simulink library "RF"  (Simulink 4.00)
values from neighbouring files (symbols this model uses):
  A = rms(interp1(f,MX,fb))    [fftbandamp.m]    (also in logfft.m = fftamp(samples, fs, f, varargin{:})/vpp; plotfft.m = fftamp(samples, fs, f, varargin{:})*2/vpp)
  P = sinc((1575.42 - f)/10.23).^2./10.23    [L1PSD.m]    (also in fftphase.m = interp1(f,PX,f0))
undefined symbols (not defined in the file or in its folder): adb, B, CA_ID, fs, j, m, N, p, Phi, Range, Rice_K, Rice_Seed, Rice_Sigma, tau_delay, z
libraries: RF x133, dspcmplx x47, com_sour x8, dspelmat x8, com_chan x4, dspbdsp x3, dspswit x3, simulink_extras x2, com_filt x2
(part 3 of 5)

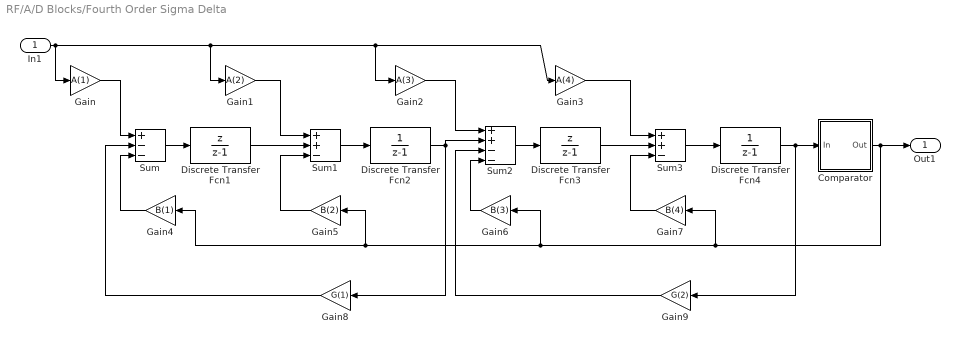
== system RF/A/D Blocks/Fourth Order Sigma Delta ==
  In1 : Inport  Port=1
  Comparator : Subsystem  mask(Comparator){L_Out=-1, H_Out=1, Bound=0}
      mask prompts: L_Out "Low Output"; H_Out "High Output"; Bound "Boundary"
      mask help: Comparator
      settings: RTWFcnNameOpts=Auto  RTWFileNameOpts=Auto
      mask Help: Outputs "low" level when the input is less than the boundary setting, and "high" when the input is above the boundary setting.
      mask Display: plot(0,0,100,100,[50,50],[0,100],[100,0],[50,50],[100,50],[70,70],[50,-0],[30,30])
  Discrete Transfer Fcn1 : DiscreteTransferFcn  Numerator=[1 0]  Denominator=[1 -1]  SampleTime=ts  Realization=auto
  Discrete Transfer Fcn2 : DiscreteTransferFcn  Numerator=[1]  Denominator=[1 -1]  SampleTime=ts  Realization=auto
  Discrete Transfer Fcn3 : DiscreteTransferFcn  Numerator=[1 0]  Denominator=[1 -1]  SampleTime=ts  Realization=auto
  Discrete Transfer Fcn4 : DiscreteTransferFcn  Numerator=[1]  Denominator=[1 -1]  SampleTime=ts  Realization=auto
  Gain : Gain  Gain=A(1)  Multiplication=Element-wise(K.*u)  SaturateOnIntegerOverflow=on
  Gain1 : Gain  Gain=A(2)  Multiplication=Element-wise(K.*u)  SaturateOnIntegerOverflow=on
  Gain2 : Gain  Gain=A(3)  Multiplication=Element-wise(K.*u)  SaturateOnIntegerOverflow=on
  Gain3 : Gain  Gain=A(4)  Multiplication=Element-wise(K.*u)  SaturateOnIntegerOverflow=on
  Gain4 : Gain  Orientation=left  Gain=B(1)  Multiplication=Element-wise(K.*u)  SaturateOnIntegerOverflow=on
  Gain5 : Gain  Orientation=left  Gain=B(2)  Multiplication=Element-wise(K.*u)  SaturateOnIntegerOverflow=on
  Gain6 : Gain  Orientation=left  Gain=B(3)  Multiplication=Element-wise(K.*u)  SaturateOnIntegerOverflow=on
  Gain7 : Gain  Orientation=left  Gain=B(4)  Multiplication=Element-wise(K.*u)  SaturateOnIntegerOverflow=on
  Gain8 : Gain  Orientation=left  Gain=G(1)  Multiplication=Element-wise(K.*u)  SaturateOnIntegerOverflow=on
  Gain9 : Gain  Orientation=left  Gain=G(2)  Multiplication=Element-wise(K.*u)  SaturateOnIntegerOverflow=on
  Sum : Sum  Inputs=+--  SaturateOnIntegerOverflow=on
  Sum1 : Sum  Inputs=++-  SaturateOnIntegerOverflow=on
  Sum2 : Sum  Inputs=++--  SaturateOnIntegerOverflow=on
  Sum3 : Sum  Inputs=++-  SaturateOnIntegerOverflow=on
  Out1 : Outport  Port=1  InitialOutput=0
  wires:
  Discrete Transfer Fcn4/1 -> Gain9/1, Comparator/1(In)
  Gain9/1 -> Sum2/3
  Gain6/1 -> Sum2/4
  Gain8/1 -> Sum/2
  Gain4/1 -> Sum/3
  Discrete Transfer Fcn2/1 -> Gain8/1, Sum2/2
  Gain2/1 -> Sum2/1
  Gain3/1 -> Sum3/1
  Gain1/1 -> Sum1/1
  Gain/1 -> Sum/1
  In1/1 -> Gain/1, Gain1/1, Gain3/1, Gain2/1
  Gain5/1 -> Sum1/3
  Gain7/1 -> Sum3/3
  Discrete Transfer Fcn3/1 -> Sum3/2
  Discrete Transfer Fcn1/1 -> Sum1/2
  Comparator/1(Out) -> Gain7/1, Gain6/1, Gain5/1, Gain4/1, Out1/1
  Sum3/1 -> Discrete Transfer Fcn4/1
  Sum/1 -> Discrete Transfer Fcn1/1
  Sum1/1 -> Discrete Transfer Fcn2/1
  Sum2/1 -> Discrete Transfer Fcn3/1

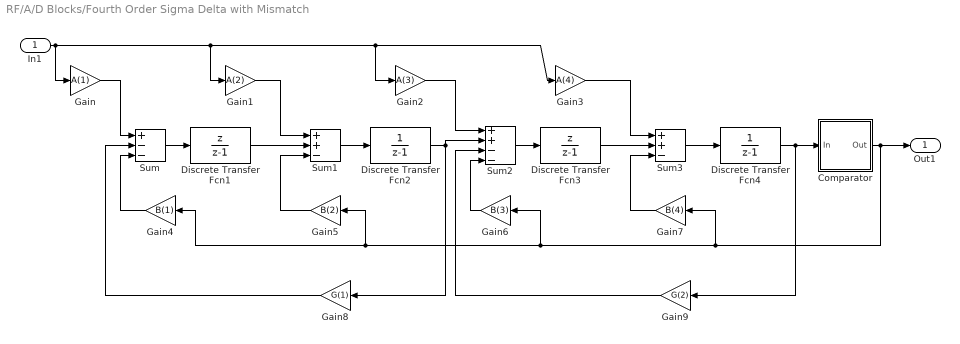
== system RF/A/D Blocks/Fourth Order Sigma Delta with Mismatch ==
  In1 : Inport  Port=1
  Comparator : Subsystem  mask(Comparator){L_Out=-1, H_Out=1, Bound=0}
      mask prompts: L_Out "Low Output"; H_Out "High Output"; Bound "Boundary"
      mask help: Comparator
      settings: RTWFcnNameOpts=Auto  RTWFileNameOpts=Auto
      mask Help: Outputs "low" level when the input is less than the boundary setting, and "high" when the input is above the boundary setting.
      mask Display: plot(0,0,100,100,[50,50],[0,100],[100,0],[50,50],[100,50],[70,70],[50,-0],[30,30])
  Discrete Transfer Fcn1 : DiscreteTransferFcn  Numerator=[1 0]  Denominator=[1 -1]  SampleTime=ts  Realization=auto
  Discrete Transfer Fcn2 : DiscreteTransferFcn  Numerator=[1]  Denominator=[1 -1]  SampleTime=ts  Realization=auto
  Discrete Transfer Fcn3 : DiscreteTransferFcn  Numerator=[1 0]  Denominator=[1 -1]  SampleTime=ts  Realization=auto
  Discrete Transfer Fcn4 : DiscreteTransferFcn  Numerator=[1]  Denominator=[1 -1]  SampleTime=ts  Realization=auto
  Gain : Gain  Gain=A(1)  Multiplication=Element-wise(K.*u)  SaturateOnIntegerOverflow=on
  Gain1 : Gain  Gain=A(2)  Multiplication=Element-wise(K.*u)  SaturateOnIntegerOverflow=on
  Gain2 : Gain  Gain=A(3)  Multiplication=Element-wise(K.*u)  SaturateOnIntegerOverflow=on
  Gain3 : Gain  Gain=A(4)  Multiplication=Element-wise(K.*u)  SaturateOnIntegerOverflow=on
  Gain4 : Gain  Orientation=left  Gain=B(1)  Multiplication=Element-wise(K.*u)  SaturateOnIntegerOverflow=on
  Gain5 : Gain  Orientation=left  Gain=B(2)  Multiplication=Element-wise(K.*u)  SaturateOnIntegerOverflow=on
  Gain6 : Gain  Orientation=left  Gain=B(3)  Multiplication=Element-wise(K.*u)  SaturateOnIntegerOverflow=on
  Gain7 : Gain  Orientation=left  Gain=B(4)  Multiplication=Element-wise(K.*u)  SaturateOnIntegerOverflow=on
  Gain8 : Gain  Orientation=left  Gain=G(1)  Multiplication=Element-wise(K.*u)  SaturateOnIntegerOverflow=on
  Gain9 : Gain  Orientation=left  Gain=G(2)  Multiplication=Element-wise(K.*u)  SaturateOnIntegerOverflow=on
  Sum : Sum  Inputs=+--  SaturateOnIntegerOverflow=on
  Sum1 : Sum  Inputs=++-  SaturateOnIntegerOverflow=on
  Sum2 : Sum  Inputs=++--  SaturateOnIntegerOverflow=on
  Sum3 : Sum  Inputs=++-  SaturateOnIntegerOverflow=on
  Out1 : Outport  Port=1  InitialOutput=0
  wires:
  Sum2/1 -> Discrete Transfer Fcn3/1
  Sum1/1 -> Discrete Transfer Fcn2/1
  Sum/1 -> Discrete Transfer Fcn1/1
  Sum3/1 -> Discrete Transfer Fcn4/1
  Comparator/1(Out) -> Out1/1, Gain4/1, Gain5/1, Gain6/1, Gain7/1
  Discrete Transfer Fcn1/1 -> Sum1/2
  Discrete Transfer Fcn3/1 -> Sum3/2
  Gain7/1 -> Sum3/3
  Gain5/1 -> Sum1/3
  In1/1 -> Gain2/1, Gain3/1, Gain1/1, Gain/1
  Gain/1 -> Sum/1
  Gain1/1 -> Sum1/1
  Gain3/1 -> Sum3/1
  Gain2/1 -> Sum2/1
  Discrete Transfer Fcn2/1 -> Sum2/2, Gain8/1
  Gain4/1 -> Sum/3
  Gain8/1 -> Sum/2
  Gain6/1 -> Sum2/4
  Gain9/1 -> Sum2/3
  Discrete Transfer Fcn4/1 -> Comparator/1(In), Gain9/1

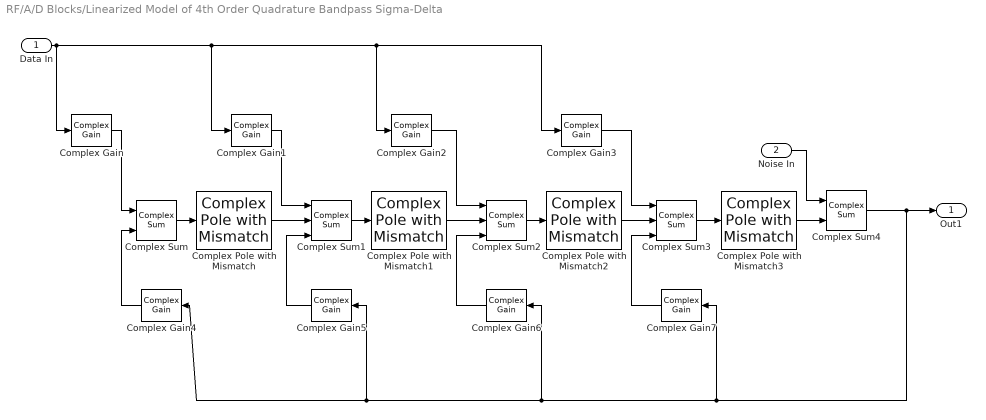
== system RF/A/D Blocks/Linearized Model of 4th Order Quadrature Bandpass Sigma-Delta ==
  Data In : Inport  Port=1
  Noise In : Inport  Port=2
  Complex Gain : RF/Complex Blocks/Complex Gain  G=a(1)+j*e(1)
  Complex Gain1 : RF/Complex Blocks/Complex Gain  G=a(2)+j*e(2)
  Complex Gain2 : RF/Complex Blocks/Complex Gain  G=a(3)+j*e(3)
  Complex Gain3 : RF/Complex Blocks/Complex Gain  G=a(4)+j*e(4)
  Complex Gain4 : RF/Complex Blocks/Complex Gain  Orientation=left  G=b(1)+j*f(1)
  Complex Gain5 : RF/Complex Blocks/Complex Gain  Orientation=left  G=b(2)+j*f(2)
  Complex Gain6 : RF/Complex Blocks/Complex Gain  Orientation=left  G=b(3)+j*f(3)
  Complex Gain7 : RF/Complex Blocks/Complex Gain  Orientation=left  G=b(4)+j*f(4)
  Complex Pole with Mismatch : RF/Complex Blocks/Complex Pole with Mismatch  c1=c1(1)  c2=c2(1)  d1=d1(1)  d2=d2(1)  ts=ts
  Complex Pole with Mismatch1 : RF/Complex Blocks/Complex Pole with Mismatch  c1=c1(2)  c2=c2(2)  d1=d1(2)  d2=d2(2)  ts=ts
  Complex Pole with Mismatch2 : RF/Complex Blocks/Complex Pole with Mismatch  c1=c1(3)  c2=c2(3)  d1=d1(3)  d2=d2(3)  ts=ts
  Complex Pole with Mismatch3 : RF/Complex Blocks/Complex Pole with Mismatch  c1=c1(4)  c2=c2(4)  d1=d1(4)  d2=d2(4)  ts=ts
  Complex Sum : dspcmplx/Complex Sum  Inputs=++
  Complex Sum1 : dspcmplx/Complex Sum  Inputs=+++
  Complex Sum2 : dspcmplx/Complex Sum  Inputs=+++
  Complex Sum3 : dspcmplx/Complex Sum  Inputs=+++
  Complex Sum4 : dspcmplx/Complex Sum  Inputs=++
  Out1 : Outport  Port=1  InitialOutput=0
  wires:
  Complex Gain4/1 -> Complex Sum/2
  Complex Pole with Mismatch/1 -> Complex Sum1/2
  Complex Sum1/1 -> Complex Pole with Mismatch1/1
  Complex Gain/1 -> Complex Sum/1
  Complex Gain1/1 -> Complex Sum1/1
  Data In/1 -> Complex Gain/1, Complex Gain1/1, Complex Gain3/1, Complex Gain2/1
  Complex Gain5/1 -> Complex Sum1/3
  Complex Sum/1 -> Complex Pole with Mismatch/1
  Complex Pole with Mismatch2/1 -> Complex Sum3/2
  Complex Pole with Mismatch1/1 -> Complex Sum2/2
  Complex Gain7/1 -> Complex Sum3/3
  Complex Gain6/1 -> Complex Sum2/3
  Complex Sum2/1 -> Complex Pole with Mismatch2/1
  Complex Gain3/1 -> Complex Sum3/1
  Complex Gain2/1 -> Complex Sum2/1
  Complex Sum3/1 -> Complex Pole with Mismatch3/1
  Complex Pole with Mismatch3/1 -> Complex Sum4/2
  Complex Sum4/1 -> Out1/1, Complex Gain7/1, Complex Gain6/1, Complex Gain5/1, Complex Gain4/1
  Noise In/1 -> Complex Sum4/1

== system RF/A/D Blocks/Second Order Simple  Lowpass  Sigma-Delta ==
  Analog_In : Inport  Port=1
  Comparator : Subsystem  mask(Comparator){L_Out=-1, H_Out=1, Bound=0}
      mask prompts: L_Out "Low Output"; H_Out "High Output"; Bound "Boundary"
      mask help: Comparator
      settings: RTWFcnNameOpts=Auto  RTWFileNameOpts=Auto
      mask Help: Outputs "low" level when the input is less than the boundary setting, and "high" when the input is above the boundary setting.
      mask Display: plot(0,0,100,100,[50,50],[0,100],[100,0],[50,50],[100,50],[70,70],[50,-0],[30,30])
  Sum : Sum  Inputs=-+  SaturateOnIntegerOverflow=on
  Sum1 : Sum  Inputs=++  SaturateOnIntegerOverflow=on
  Sum2 : Sum  Inputs=-+  SaturateOnIntegerOverflow=on
  Sum3 : Sum  Inputs=++  SaturateOnIntegerOverflow=on
  Unit Delay : UnitDelay  Orientation=left  X0=1  SampleTime=1/fs
  Unit Delay1 : UnitDelay  X0=1  SampleTime=1/fs
  Data_Out : Outport  Port=1  InitialOutput=0
  wires:
  Comparator/1(Out) -> Sum2/1, Sum/1, Data_Out/1
  Unit Delay1/1 -> Comparator/1(In), Sum3/2
  Sum2/1 -> Sum3/1
  Sum3/1 -> Unit Delay1/1
  Sum1/1 -> Sum2/2, Unit Delay/1
  Unit Delay/1 -> Sum1/2
  Analog_In/1 -> Sum/2
  Sum/1 -> Sum1/1

== system RF/A/D Blocks/Second-Order Integrator ==
  Data In : Inport  Port=1
  Discrete Filter : DiscreteFilter  Numerator=[1 zeros(1,N-1) -1]  Denominator=[1 -1]  SampleTime=1/fs  Realization=auto
  Discrete Filter1 : DiscreteFilter  Numerator=[1 zeros(1,N-1) -1]  Denominator=[1 -1]  SampleTime=1/fs  Realization=auto
  Gain : Gain  Gain=1/N  Multiplication=Element-wise(K.*u)  SaturateOnIntegerOverflow=on
  Gain1 : Gain  Gain=1/N  Multiplication=Element-wise(K.*u)  SaturateOnIntegerOverflow=on
  Data Out : Outport  Port=1  InitialOutput=0
  wires:
  Gain1/1 -> Data Out/1
  Data In/1 -> Discrete Filter/1
  Discrete Filter/1 -> Gain/1
  Discrete Filter1/1 -> Gain1/1
  Gain/1 -> Discrete Filter1/1

== system RF/A/D Blocks/Simple BandPass Sigma-Delta ==
  Analog_In : Inport  Port=1
  Comparator : RF/Circuit Models/Comparator  L_Out=-1  H_Out=1  Bound=0
  Discrete Transfer Fcn : DiscreteTransferFcn  Numerator=[-1]  Denominator="[1  0 1]"  SampleTime=1/fs  Realization=auto
  Sum : Sum  Inputs=-+  SaturateOnIntegerOverflow=on
  Data_Out : Outport  Port=1  InitialOutput=0
  wires:
  Discrete Transfer Fcn/1 -> Comparator/1
  Comparator/1 -> Sum/1, Data_Out/1
  Sum/1 -> Discrete Transfer Fcn/1
  Analog_In/1 -> Sum/2

== system RF/A/D Blocks/Simple Lowpass  Sigma-Delta ==
  Analog_In : Inport  Port=1
  Comparator : Subsystem  mask(Comparator){L_Out=-1, H_Out=1, Bound=0}
      mask prompts: L_Out "Low Output"; H_Out "High Output"; Bound "Boundary"
      mask help: Comparator
      settings: RTWFcnNameOpts=Auto  RTWFileNameOpts=Auto
      mask Help: Outputs "low" level when the input is less than the boundary setting, and "high" when the input is above the boundary setting.
      mask Display: plot(0,0,100,100,[50,50],[0,100],[100,0],[50,50],[100,50],[70,70],[50,-0],[30,30])
  Sum : Sum  Inputs=-+  SaturateOnIntegerOverflow=on
  Sum1 : Sum  Inputs=++  SaturateOnIntegerOverflow=on
  Unit Delay : UnitDelay  X0=1  SampleTime=1/fs
  Data_Out : Outport  Port=1  InitialOutput=0
  wires:
  Analog_In/1 -> Sum/2
  Comparator/1(Out) -> Data_Out/1, Sum/1
  Sum/1 -> Sum1/1
  Sum1/1 -> Unit Delay/1
  Unit Delay/1 -> Comparator/1(In), Sum1/2

== system RF/A/D Blocks/Simple Quadrature BandPass Sigma-Delta ==
  Comp_In : Inport  Port=1
  Complex Quantizer1 : RF/Complex Blocks/Complex Quantizer  L_Out_C=-1  H_Out_C=1  Bound_C=0
  Complex Resonator : Subsystem
      settings: RTWFcnNameOpts=Auto  RTWFileNameOpts=Auto
      mask Type: Complex Resonator
      mask Display: disp('Resonator')
  Complex Sum : dspcmplx/Complex Sum  Inputs=-+
  Data Out : Outport  Port=1  InitialOutput=0
  wires:
  Complex Sum/1 -> Complex Resonator/1(In1)
  Comp_In/1 -> Complex Sum/2
  Complex Quantizer1/1 -> Complex Sum/1, Data Out/1
  Complex Resonator/1(Out1) -> Complex Quantizer1/1

== system RF/A/D Blocks/Third-Order Integrator ==
  Data In : Inport  Port=1
  Discrete Filter : DiscreteFilter  Numerator=[1 zeros(1,N-1) -1]  Denominator=[1 -1]  SampleTime=1/fs  Realization=auto
  Discrete Filter1 : DiscreteFilter  Numerator=[1 zeros(1,N-1) -1]  Denominator=[1 -1]  SampleTime=1/fs  Realization=auto
  Discrete Filter2 : DiscreteFilter  Numerator=[1 zeros(1,N-1) -1]  Denominator=[1 -1]  SampleTime=1/fs  Realization=auto
  Gain : Gain  Gain=1/N  Multiplication=Element-wise(K.*u)  SaturateOnIntegerOverflow=on
  Gain1 : Gain  Gain=1/N  Multiplication=Element-wise(K.*u)  SaturateOnIntegerOverflow=on
  Gain2 : Gain  Gain=1/N  Multiplication=Element-wise(K.*u)  SaturateOnIntegerOverflow=on
  Data Out : Outport  Port=1  InitialOutput=0
  wires:
  Gain2/1 -> Data Out/1
  Gain1/1 -> Discrete Filter2/1
  Discrete Filter2/1 -> Gain2/1
  Data In/1 -> Discrete Filter/1
  Discrete Filter/1 -> Gain/1
  Discrete Filter1/1 -> Gain1/1
  Gain/1 -> Discrete Filter1/1

== system RF/Circuit Models/Clock  with Jitter ==
  Clock : Clock
      settings: DisplayTime=off  Decimation=10
  Comparator with Hysteresis : RF/Circuit Models/Comparator with Hysteresis  L_Out=VLow  H_Out=VHigh  Bound=sin(pi*(0.5-DCycle))  NPeak=PError*pi/50
  Fcn : Fcn  Expr=sin(2*pi*f0*u+Phase0)
  Gaussian noise generator : com_sour/Gaussian noise generator  m=0  d=(PError/f0/300)^2  s=Seed
  Sum : Sum  Inputs=++  SaturateOnIntegerOverflow=on
  Out1 : Outport  Port=1  InitialOutput=0
  wires:
  Fcn/1 -> Comparator with Hysteresis/1
  Comparator with Hysteresis/1 -> Out1/1
  Sum/1 -> Fcn/1
  Clock/1 -> Sum/1
  Gaussian noise generator/1 -> Sum/2

== system RF/Circuit Models/Clock  without Jitter ==
  Clock : Clock
      settings: DisplayTime=off  Decimation=10
  Comparator with Hysteresis1 : RF/Circuit Models/Comparator with Hysteresis  L_Out=VLow  H_Out=VHigh  Bound=sin(pi*(0.5-DCycle))  NPeak=PError*pi/50
  Fcn : Fcn  Expr=sin(2*pi*f0*u+Phase0)
  Out1 : Outport  Port=1  InitialOutput=0
  wires:
  Fcn/1 -> Comparator with Hysteresis1/1
  Comparator with Hysteresis1/1 -> Out1/1
  Clock/1 -> Fcn/1

== system RF/Circuit Models/Comparator ==
  In : Inport  Port=1
  Relay : Relay  OnSwitchValue=Bound  OffSwitchValue=Bound  OnOutputValue=H_Out  OffOutputValue=L_Out
  Out : Outport  Port=1  InitialOutput=0
  wires:
  Relay/1 -> Out/1
  In/1 -> Relay/1

== system RF/Circuit Models/Comparator with Hysteresis ==
  In : Inport  Port=1
  Relay : Relay  OnSwitchValue=Bound + NPeak  OffSwitchValue=Bound - NPeak  OnOutputValue=H_Out  OffOutputValue=L_Out
  Out : Outport  Port=1  InitialOutput=0
  wires:
  In/1 -> Relay/1
  Relay/1 -> Out/1

== system RF/Circuit Models/Non-Ideal Mixer ==
  RF : Inport  Port=1
  LO : Inport  Port=2
  Compression : RF/Model Nonidealities/Compression  V1dB=V1dB
  Flicker Noise : RF/Model Nonidealities/Flicker Noise  f0=f0  N0=N0  fm=fm  numtaps=numtaps  Seed=Fseed
  Nonlinear TF : RF/Model Nonidealities/Nonlinear TF  Gain1=Gain1  IIP2=IIP2  IIP3=IIP3
  Product : Product  Inputs=2  Multiplication=Element-wise(.*)  SaturateOnIntegerOverflow=on
  Saturation : Saturate  UpperLimit=1  LowerLimit=-1  LinearizeAsGain=on
  Slew Rate : RateLimiter  RisingSlewLimit=2*pi*fmax*2  FallingSlewLimit=-2*pi*fmax*2
  Sum : Sum  Inputs=++  SaturateOnIntegerOverflow=on
  White Noise : com_chan/AWGN channel  m=0  d=AWGNVRMS^2  s=SeedAWGN
  IF : Outport  Port=1  InitialOutput=0
  wires:
  RF/1 -> Product/1
  LO/1 -> Product/2
  Nonlinear TF/1 -> White Noise/1
  Product/1 -> Nonlinear TF/1
  White Noise/1 -> Sum/1
  Flicker Noise/1 -> Sum/2
  Compression/1 -> Slew Rate/1
  Slew Rate/1 -> Saturation/1
  Saturation/1 -> IF/1
  Sum/1 -> Compression/1

== system RF/Circuit Models/Non-Ideal  LNA ==
  In1 : Inport  Port=1
  Compression : RF/Model Nonidealities/Compression  V1dB=V1dB
  Flicker Noise : RF/Model Nonidealities/Flicker Noise  f0=f0  N0=N0  fm=fm  numtaps=numtaps  Seed=FSeed
  Nonlinear TF : RF/Model Nonidealities/Nonlinear TF  Gain1=Gain1  IIP2=IIP2  IIP3=IIP3
  Saturation : Saturate  UpperLimit=1  LowerLimit=-1  LinearizeAsGain=on
  Slew Rate : RateLimiter  RisingSlewLimit=2*pi*fmax*2  FallingSlewLimit=-2*pi*fmax*2
  Sum : Sum  Inputs=++  SaturateOnIntegerOverflow=on
  White Noise : com_chan/AWGN channel  m=0  d=AWGNVRMS^2  s=SeedAWGN
  Out1 : Outport  Port=1  InitialOutput=0
  wires:
  Nonlinear TF/1 -> White Noise/1
  In1/1 -> Nonlinear TF/1
  White Noise/1 -> Sum/1
  Flicker Noise/1 -> Sum/2
  Compression/1 -> Slew Rate/1
  Slew Rate/1 -> Saturation/1
  Saturation/1 -> Out1/1
  Sum/1 -> Compression/1

== system RF/Circuit Models/Quadrature Oscillator ==
  I : Sin  Amplitude=(1+AE)*A  Frequency=f0*2*pi  Phase=Phi + (pi/2 + PhiE)  SampleTime=0
  Q : Sin  Amplitude=1*A  Frequency=f0*2*pi  Phase=Phi  SampleTime=0
  Out1 : Outport  Port=1  InitialOutput=0
  Out2 : Outport  Port=2  InitialOutput=0
  wires:
  Q/1 -> Out2/1
  I/1 -> Out1/1

== system RF/Circuit Models/Simple Non-Ideal Mixer ==
  RF : Inport  Port=1
  LO : Inport  Port=2
  Nonlinear TF : RF/Model Nonidealities/Nonlinear TF  Gain1=Gain1  IIP2=IIP2  IIP3=IIP3
  Product : Product  Inputs=2  Multiplication=Element-wise(.*)  SaturateOnIntegerOverflow=on
  White Noise : com_chan/AWGN channel  m=0  d=AWGNVRMS^2  s=SeedAWGN
  IF : Outport  Port=1  InitialOutput=0
  wires:
  White Noise/1 -> IF/1
  RF/1 -> Product/1
  LO/1 -> Product/2
  Nonlinear TF/1 -> White Noise/1
  Product/1 -> Nonlinear TF/1

== system RF/Circuit Models/Simple Non-Ideal  LNA ==
  In1 : Inport  Port=1
  Nonlinear TF : RF/Model Nonidealities/Nonlinear TF  Gain1=Gain1  IIP2=IIP2  IIP3=IIP3
  White Noise : com_chan/AWGN channel  m=0  d=AWGNVRMS^2  s=SeedAWGN
  Out1 : Outport  Port=1  InitialOutput=0
  wires:
  White Noise/1 -> Out1/1
  Nonlinear TF/1 -> White Noise/1
  In1/1 -> Nonlinear TF/1

== system RF/Complex Blocks/Complex Gain ==
  In1 : Inport  Port=1
  Complex Constant : dspcmplx/Complex Constant  val=G
  Complex Multiply : dspcmplx/Complex Multiply
  Out1 : Outport  Port=1  InitialOutput=0
  wires:
  Complex Constant/1 -> Complex Multiply/2
  In1/1 -> Complex Multiply/1
  Complex Multiply/1 -> Out1/1

== system RF/Complex Blocks/Complex Quantizer ==
  In1 : Inport  Port=1
  Comparator : RF/Circuit Models/Comparator  L_Out=L_Out_C  H_Out=H_Out_C  Bound=Bound_C
  Comparator1 : RF/Circuit Models/Comparator  L_Out=L_Out_C  H_Out=H_Out_C  Bound=Bound_C
  Join : dspcmplx/Join
  Split : dspcmplx/Split
  Out1 : Outport  Port=1  InitialOutput=0
  wires:
  Split/1 -> Comparator/1
  Split/2 -> Comparator1/1
  Comparator/1 -> Join/1
  Comparator1/1 -> Join/2
  Join/1 -> Out1/1
  In1/1 -> Split/1

== system RF/Complex Blocks/Complex Unit Delay ==
  In1 : Inport  Port=1
  Join : dspcmplx/Join
  Split : dspcmplx/Split
  Unit Delay : UnitDelay  X0=icr  SampleTime=ts
  Unit Delay1 : UnitDelay  X0=ici  SampleTime=ts
  Out1 : Outport  Port=1  InitialOutput=0
  wires:
  In1/1 -> Split/1
  Join/1 -> Out1/1
  Split/2 -> Unit Delay1/1
  Split/1 -> Unit Delay/1
  Unit Delay1/1 -> Join/2
  Unit Delay/1 -> Join/1

== system RF/Complex Blocks/Complex  Continuous Pole ==
  Comp In : Inport  Port=1
  Gain1 : Gain  Orientation=left  Gain=c  Multiplication=Element-wise(K.*u)  SaturateOnIntegerOverflow=on
  Gain2 : Gain  Orientation=left  Gain=d  Multiplication=Element-wise(K.*u)  SaturateOnIntegerOverflow=on
  Gain3 : Gain  Orientation=left  Gain=c  Multiplication=Element-wise(K.*u)  SaturateOnIntegerOverflow=on
  Gain4 : Gain  Orientation=left  Gain=d  Multiplication=Element-wise(K.*u)  SaturateOnIntegerOverflow=on
  Join : dspcmplx/Join
  Split : dspcmplx/Split
  Sum : Sum  Inputs=+++  SaturateOnIntegerOverflow=on
  Sum1 : Sum  Inputs=++-  SaturateOnIntegerOverflow=on
  Transfer Fcn : TransferFcn  Numerator=[1]  Denominator=[1 0]  Realization=auto  AbsoluteTolerance=auto
  Transfer Fcn1 : TransferFcn  Numerator=[1]  Denominator=[1 0]  Realization=auto  AbsoluteTolerance=auto
  Comp Out : Outport  Port=1  InitialOutput=0
  wires:
  Comp In/1 -> Split/1
  Gain1/1 -> Sum/1
  Split/2 -> Sum/2
  Split/1 -> Sum1/2
  Gain3/1 -> Sum1/3
  Join/1 -> Comp Out/1
  Sum/1 -> Transfer Fcn/1
  Sum1/1 -> Transfer Fcn1/1
  Transfer Fcn/1 -> Gain3/1, Join/2, Gain2/1
  Transfer Fcn1/1 -> Gain1/1, Join/1, Gain4/1
  Gain2/1 -> Sum/3
  Gain4/1 -> Sum1/1

== system RF/Complex Blocks/Complex Continuous Pole with Mismatch  ==
  Comp In : Inport  Port=1
  Gain1 : Gain  Orientation=left  Gain=c2  Multiplication=Element-wise(K.*u)  SaturateOnIntegerOverflow=on
  Gain2 : Gain  Orientation=left  Gain=d2  Multiplication=Element-wise(K.*u)  SaturateOnIntegerOverflow=on
  Gain3 : Gain  Orientation=left  Gain=c1  Multiplication=Element-wise(K.*u)  SaturateOnIntegerOverflow=on
  Gain4 : Gain  Orientation=left  Gain=d1  Multiplication=Element-wise(K.*u)  SaturateOnIntegerOverflow=on
  Join : dspcmplx/Join
  Split : dspcmplx/Split
  Sum : Sum  Inputs=+++  SaturateOnIntegerOverflow=on
  Sum1 : Sum  Inputs=++-  SaturateOnIntegerOverflow=on
  Transfer Fcn : TransferFcn  Numerator=[1]  Denominator=[1 0]  Realization=auto  AbsoluteTolerance=auto
  Transfer Fcn1 : TransferFcn  Numerator=[1]  Denominator=[1 0]  Realization=auto  AbsoluteTolerance=auto
  Comp Out : Outport  Port=1  InitialOutput=0
  wires:
  Gain4/1 -> Sum1/1
  Gain2/1 -> Sum/3
  Transfer Fcn1/1 -> Gain4/1, Join/1, Gain1/1
  Transfer Fcn/1 -> Gain2/1, Join/2, Gain3/1
  Sum1/1 -> Transfer Fcn1/1
  Sum/1 -> Transfer Fcn/1
  Join/1 -> Comp Out/1
  Gain3/1 -> Sum1/3
  Split/1 -> Sum1/2
  Split/2 -> Sum/2
  Gain1/1 -> Sum/1
  Comp In/1 -> Split/1

== system RF/Complex Blocks/Complex Pole ==
  Comp In : Inport  Port=1
  Discrete Transfer Fcn : DiscreteTransferFcn  Numerator=[1]  Denominator=[1 -1]  SampleTime=ts  Realization=auto
  Discrete Transfer Fcn1 : DiscreteTransferFcn  Numerator=[1]  Denominator=[1 -1]  SampleTime=ts  Realization=auto
  Gain : Gain  Orientation=left  Gain=d  Multiplication=Element-wise(K.*u)  SaturateOnIntegerOverflow=on
  Gain1 : Gain  Orientation=left  Gain=c  Multiplication=Element-wise(K.*u)  SaturateOnIntegerOverflow=on
  Gain2 : Gain  Orientation=left  Gain=c  Multiplication=Element-wise(K.*u)  SaturateOnIntegerOverflow=on
  Gain3 : Gain  Orientation=left  Gain=d  Multiplication=Element-wise(K.*u)  SaturateOnIntegerOverflow=on
  Join : dspcmplx/Join
  Split : dspcmplx/Split
  Sum : Sum  Inputs=++-  SaturateOnIntegerOverflow=on
  Sum1 : Sum  Inputs=+++  SaturateOnIntegerOverflow=on
  Comp Out : Outport  Port=1  InitialOutput=0
  wires:
  Sum1/1 -> Discrete Transfer Fcn1/1
  Sum/1 -> Discrete Transfer Fcn/1
  Gain1/1 -> Sum/3
  Gain/1 -> Sum/1
  Gain2/1 -> Sum1/1
  Gain3/1 -> Sum1/3
  Discrete Transfer Fcn1/1 -> Gain1/1, Gain3/1, Join/2
  Discrete Transfer Fcn/1 -> Gain2/1, Gain/1, Join/1
  Comp In/1 -> Split/1
  Split/1 -> Sum/2
  Split/2 -> Sum1/2
  Join/1 -> Comp Out/1

== system RF/Complex Blocks/Complex Pole with Mismatch ==
  Comp In : Inport  Port=1
  Discrete Transfer Fcn : DiscreteTransferFcn  Numerator=[1]  Denominator=[1 -1]  SampleTime=ts  Realization=auto
  Discrete Transfer Fcn1 : DiscreteTransferFcn  Numerator=[1]  Denominator=[1 -1]  SampleTime=ts  Realization=auto
  Gain : Gain  Orientation=left  Gain=d1  Multiplication=Element-wise(K.*u)  SaturateOnIntegerOverflow=on
  Gain1 : Gain  Orientation=left  Gain=c1  Multiplication=Element-wise(K.*u)  SaturateOnIntegerOverflow=on
  Gain2 : Gain  Orientation=left  Gain=c2  Multiplication=Element-wise(K.*u)  SaturateOnIntegerOverflow=on
  Gain3 : Gain  Orientation=left  Gain=d2  Multiplication=Element-wise(K.*u)  SaturateOnIntegerOverflow=on
  Join : dspcmplx/Join
  Split : dspcmplx/Split
  Sum : Sum  Inputs=++-  SaturateOnIntegerOverflow=on
  Sum1 : Sum  Inputs=+++  SaturateOnIntegerOverflow=on
  Comp Out : Outport  Port=1  InitialOutput=0
  wires:
  Sum1/1 -> Discrete Transfer Fcn1/1
  Sum/1 -> Discrete Transfer Fcn/1
  Gain1/1 -> Sum/3
  Gain/1 -> Sum/1
  Gain2/1 -> Sum1/1
  Gain3/1 -> Sum1/3
  Discrete Transfer Fcn1/1 -> Gain1/1, Gain3/1, Join/2
  Discrete Transfer Fcn/1 -> Gain2/1, Gain/1, Join/1
  Comp In/1 -> Split/1
  Split/1 -> Sum/2
  Split/2 -> Sum1/2
  Join/1 -> Comp Out/1

== system RF/Complex Blocks/Complex Random  Number ==
  Join : dspcmplx/Join
  Random Number : RandomNumber  Mean=Mean  Variance=Sigma  Seed=Seeds(2)  SampleTime=0
  Random Number1 : RandomNumber  Mean=Mean  Variance=Sigma  Seed=Seeds(1)  SampleTime=0
  Out1 : Outport  Port=1  InitialOutput=0
  wires:
  Join/1 -> Out1/1
  Random Number1/1 -> Join/1
  Random Number/1 -> Join/2

== system RF/Filters/Butterworth BP Filter ==
  In1 : Inport  Port=1
  Butterworth BP Filter : ZeroPole  Zeros=z  Poles=p  Gain=k  AbsoluteTolerance=auto
  Out1 : Outport  Port=1  InitialOutput=0
  wires:
  In1/1 -> Butterworth BP Filter/1
  Butterworth BP Filter/1 -> Out1/1

== system RF/Filters/Butterworth BP Filter with Mismatch ==
  In1 : Inport  Port=1
  Butterworth BP Filter : ZeroPole  Zeros=z  Poles=p  Gain=k  AbsoluteTolerance=auto
  Out1 : Outport  Port=1  InitialOutput=0
  wires:
  Butterworth BP Filter/1 -> Out1/1
  In1/1 -> Butterworth BP Filter/1

== system RF/Filters/Butterworth BS Filter ==
  In1 : Inport  Port=1
  Butterworth BS Filter : ZeroPole  Zeros=z  Poles=p  Gain=k  AbsoluteTolerance=auto
  Out1 : Outport  Port=1  InitialOutput=0
  wires:
  Butterworth BS Filter/1 -> Out1/1
  In1/1 -> Butterworth BS Filter/1

== system RF/Filters/Butterworth BS Filter with Mismatch ==
  In1 : Inport  Port=1
  Butterworth BS Filter : ZeroPole  Zeros=z  Poles=p  Gain=k  AbsoluteTolerance=auto
  Out1 : Outport  Port=1  InitialOutput=0
  wires:
  In1/1 -> Butterworth BS Filter/1
  Butterworth BS Filter/1 -> Out1/1

== system RF/Filters/Butterworth HP Filter ==
  In1 : Inport  Port=1
  Butterworth HP Filter : ZeroPole  Zeros=z  Poles=p  Gain=k  AbsoluteTolerance=auto
  Out1 : Outport  Port=1  InitialOutput=0
  wires:
  Butterworth HP Filter/1 -> Out1/1
  In1/1 -> Butterworth HP Filter/1

== system RF/Filters/Butterworth HP Filter with Mismatch ==
  In1 : Inport  Port=1
  Butterworth HP Filter : ZeroPole  Zeros=z  Poles=p  Gain=k  AbsoluteTolerance=auto
  Out1 : Outport  Port=1  InitialOutput=0
  wires:
  In1/1 -> Butterworth HP Filter/1
  Butterworth HP Filter/1 -> Out1/1

== system RF/Filters/Butterworth LP Filter ==
  In1 : Inport  Port=1
  Butterworth LP Filter : ZeroPole  Zeros=z  Poles=p  Gain=k  AbsoluteTolerance=auto
  Out1 : Outport  Port=1  InitialOutput=0
  wires:
  In1/1 -> Butterworth LP Filter/1
  Butterworth LP Filter/1 -> Out1/1

== system RF/Filters/Butterworth LP Filter with Mismatch ==
  In1 : Inport  Port=1
  Butterworth LP Filter : ZeroPole  Zeros=z  Poles=p  Gain=k  AbsoluteTolerance=auto
  Out1 : Outport  Port=1  InitialOutput=0
  wires:
  Butterworth LP Filter/1 -> Out1/1
  In1/1 -> Butterworth LP Filter/1

== system RF/Filters/Chebychev Type I BP Filter ==
  In1 : Inport  Port=1
  Chebychev Type I BP Filter : ZeroPole  Zeros=z  Poles=p  Gain=k  AbsoluteTolerance=auto
  Out1 : Outport  Port=1  InitialOutput=0
  wires:
  Chebychev Type I BP Filter/1 -> Out1/1
  In1/1 -> Chebychev Type I BP Filter/1

== system RF/Filters/Chebychev Type I BP Filter with Mismatch ==
  In1 : Inport  Port=1
  Chebychev Type I BP Filter : ZeroPole  Zeros=z  Poles=p  Gain=k  AbsoluteTolerance=auto
  Out1 : Outport  Port=1  InitialOutput=0
  wires:
  In1/1 -> Chebychev Type I BP Filter/1
  Chebychev Type I BP Filter/1 -> Out1/1

== system RF/Filters/Chebychev Type I BS Filter ==
  In1 : Inport  Port=1
  Chebychev Type I BS Filter : ZeroPole  Zeros=z  Poles=p  Gain=k  AbsoluteTolerance=auto
  Out1 : Outport  Port=1  InitialOutput=0
  wires:
  Chebychev Type I BS Filter/1 -> Out1/1
  In1/1 -> Chebychev Type I BS Filter/1

== system RF/Filters/Chebychev Type I BS Filter with Mismatch ==
  In1 : Inport  Port=1
  Chebychev Type I BS Filter : ZeroPole  Zeros=z  Poles=p  Gain=k  AbsoluteTolerance=auto
  Out1 : Outport  Port=1  InitialOutput=0
  wires:
  In1/1 -> Chebychev Type I BS Filter/1
  Chebychev Type I BS Filter/1 -> Out1/1

== system RF/Filters/Chebychev Type I HP Filter ==
  In1 : Inport  Port=1
  Chebychev Type I HP Filter : ZeroPole  Zeros=z  Poles=p  Gain=k  AbsoluteTolerance=auto
  Out1 : Outport  Port=1  InitialOutput=0
  wires:
  In1/1 -> Chebychev Type I HP Filter/1
  Chebychev Type I HP Filter/1 -> Out1/1

== system RF/Filters/Chebychev Type I HP Filter with Mismatch ==
  In1 : Inport  Port=1
  Chebychev Type I HP Filter : ZeroPole  Zeros=z  Poles=p  Gain=k  AbsoluteTolerance=auto
  Out1 : Outport  Port=1  InitialOutput=0
  wires:
  Chebychev Type I HP Filter/1 -> Out1/1
  In1/1 -> Chebychev Type I HP Filter/1

== system RF/Filters/Chebychev Type I LP Filter ==
  In1 : Inport  Port=1
  Chebychev Type I LP Filter : ZeroPole  Zeros=z  Poles=p  Gain=k  AbsoluteTolerance=auto
  Out1 : Outport  Port=1  InitialOutput=0
  wires:
  Chebychev Type I LP Filter/1 -> Out1/1
  In1/1 -> Chebychev Type I LP Filter/1

== system RF/Filters/Chebychev Type I LP Filter with Mismatch ==
  In1 : Inport  Port=1
  Chebychev Type I LP Filter : ZeroPole  Zeros=z  Poles=p  Gain=k  AbsoluteTolerance=auto
  Out1 : Outport  Port=1  InitialOutput=0
  wires:
  In1/1 -> Chebychev Type I LP Filter/1
  Chebychev Type I LP Filter/1 -> Out1/1

== system RF/Filters/Complex  Image-Reject  Filter ==
  In : Inport  Port=1
  Complex Gain : RF/Complex Blocks/Complex Gain  G=A
  Complex  Continuous Pole : RF/Complex Blocks/Complex  Continuous Pole  d=d(1)  c=c(1)
  Complex  Continuous Pole1 : RF/Complex Blocks/Complex  Continuous Pole  d=d(2)  c=c(2)
  Complex  Continuous Pole2 : RF/Complex Blocks/Complex  Continuous Pole  d=d(3)  c=c(3)
  Complex  Continuous Pole3 : RF/Complex Blocks/Complex  Continuous Pole  d=d(4)  c=c(4)
  Out : Outport  Port=1  InitialOutput=0
  wires:
  Complex  Continuous Pole/1 -> Complex  Continuous Pole1/1
  Complex  Continuous Pole1/1 -> Complex  Continuous Pole2/1
  Complex  Continuous Pole2/1 -> Complex  Continuous Pole3/1
  Complex  Continuous Pole3/1 -> Out/1
  Complex Gain/1 -> Complex  Continuous Pole/1
  In/1 -> Complex Gain/1

== system RF/Filters/Complex  Image-Reject  Filter with Mismatch ==
  In : Inport  Port=1
  Complex Gain : RF/Complex Blocks/Complex Gain  G=A
  "Complex Continuous Pole with Mismatch " : RF/Complex Blocks/Complex Continuous Pole with Mismatch   c1=c1(1)  c2=c2(1)  d1=d1(1)  d2=d2(1)
  Complex Continuous Pole with Mismatch 1 : RF/Complex Blocks/Complex Continuous Pole with Mismatch   c1=c1(2)  c2=c2(2)  d1=d1(2)  d2=d2(2)
  Complex Continuous Pole with Mismatch 2 : RF/Complex Blocks/Complex Continuous Pole with Mismatch   c1=c1(3)  c2=c2(3)  d1=d1(3)  d2=d2(3)
  Complex Continuous Pole with Mismatch 3 : RF/Complex Blocks/Complex Continuous Pole with Mismatch   c1=c1(4)  c2=c2(4)  d1=d1(4)  d2=d2(4)
  Out : Outport  Port=1  InitialOutput=0
  wires:
  In/1 -> Complex Gain/1
  Complex Gain/1 -> "Complex Continuous Pole with Mismatch "/1
  "Complex Continuous Pole with Mismatch "/1 -> Complex Continuous Pole with Mismatch 1/1
  Complex Continuous Pole with Mismatch 1/1 -> Complex Continuous Pole with Mismatch 2/1
  Complex Continuous Pole with Mismatch 3/1 -> Out/1
  Complex Continuous Pole with Mismatch 2/1 -> Complex Continuous Pole with Mismatch 3/1

== system RF/Filters/RF Filter ==
  In1 : Inport  Port=1
  Transfer Fcn : TransferFcn  Numerator=num  Denominator=denom  Realization=auto  AbsoluteTolerance=auto
  Out1 : Outport  Port=1  InitialOutput=0
  wires:
  In1/1 -> Transfer Fcn/1
  Transfer Fcn/1 -> Out1/1

== system RF/GPS Blocks/C/A Code, 1.023MHz ==
  note: C/A Code Generator
  Adder : Logic  Operator=XOR  Inputs=3
  CA ID : Constant  Value=CA_PRN_ID
  Look-Up Table : Lookup  InputValues=[1:32]  OutputValues=[2;3;4;5;1;2;1;2;3;2;3;5;6;7;8;9;1;2;3;4;5;6;1;4;5;6;7;8;1;2;3;4]
  Look-Up Table1 : Lookup  InputValues=[1:32]  OutputValues=[6;7;8;9;9;10;8;9;10;3;4;6;7;8;9;10;4;5;6;7;8;9;3;6;7;8;9;10;6;7;8;9]
  PN1 : Subsystem  mask(PN(10) Sequence [3,10]){}
      mask help: Pseudo Noise Sequence (M=2^10 - 1, Feedback[3,10])
      mask init:
      | [x,y]=srcsicon(5);
      settings: RTWFcnNameOpts=Auto  RTWFileNameOpts=Auto
      mask Help: Maximal length pseudo-noise sequence with 10 memory elements.  Feedback is from taps 3 and 10.  Only the 10th tap is output.
      mask Display: plot(0,0,100,100,x,y);disp('PN Sequence ')
  PN2 : Subsystem  mask(PN(10) Sequence [2,3,6,8,9,10]){}
      mask help: Pseudo Noise Sequence (M=2^10 - 1, Feedback[2,3,6,8,9,10])
      mask init:
      | [x,y]=srcsicon(5);
      settings: RTWFcnNameOpts=Auto  RTWFileNameOpts=Auto
      mask Help: Maximal length pseudo-noise sequence with 10 memory elements.  Feedback is from taps 2, 3, 6, 8, 9,  and 10.  All phases are output.
      mask Display: plot(0,0,100,100,x,y);disp('PN Sequence\nAll Phases')
  Phase 1  Select : MultiPortSwitch  Inputs=10
  Phase 2 Select : MultiPortSwitch  Inputs=10
  Out1 : Outport  Port=1  InitialOutput=0
  wires:
  Adder/1 -> Out1/1
  Phase 2 Select/1 -> Adder/3
  PN1/1(Tap10) -> Adder/1
  Phase 1  Select/1 -> Adder/2
  PN2/10(Tap10) -> Phase 2 Select/11, Phase 1  Select/11
  PN2/9(Tap9) -> Phase 2 Select/10, Phase 1  Select/10
  PN2/8(Tap8) -> Phase 2 Select/9, Phase 1  Select/9
  PN2/7(Tap7) -> Phase 2 Select/8, Phase 1  Select/8
  PN2/6(Tap6) -> Phase 2 Select/7, Phase 1  Select/7
  PN2/5(Tap5) -> Phase 2 Select/6, Phase 1  Select/6
  PN2/4(Tap4) -> Phase 2 Select/5, Phase 1  Select/5
  PN2/3(Tap3) -> Phase 2 Select/4, Phase 1  Select/4
  PN2/2(Tap2) -> Phase 2 Select/3, Phase 1  Select/3
  PN2/1(Tap1) -> Phase 2 Select/2, Phase 1  Select/2
  Look-Up Table1/1 -> Phase 2 Select/1
  Look-Up Table/1 -> Phase 1  Select/1
  CA ID/1 -> Look-Up Table/1, Look-Up Table1/1

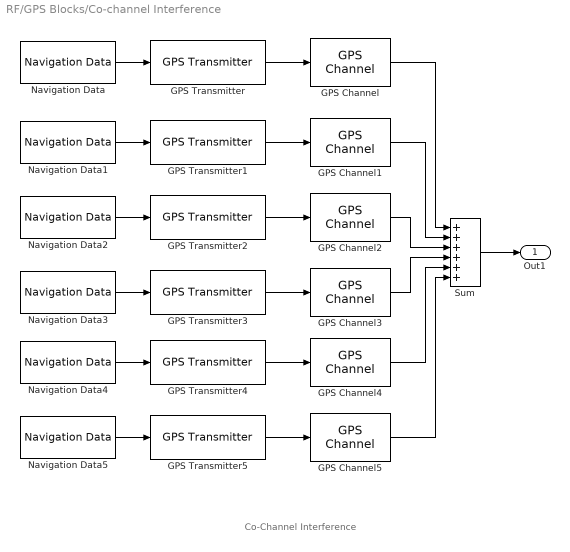
== system RF/GPS Blocks/Co-channel Interference ==
  note: Co-Channel Interference
  GPS Channel : RF/GPS Blocks/GPS Channel  Rice_Seed=Rice_Seeds(1)  tau_delay=taus_delay(1)  AWGN_Seed=AWGN_Seeds(1)  d=d(1)  tau=taus(1)
  GPS Channel1 : RF/GPS Blocks/GPS Channel  Rice_Seed=Rice_Seeds(2)  tau_delay=taus_delay(2)  AWGN_Seed=AWGN_Seeds(2)  d=d(2)  tau=taus(2)
  GPS Channel2 : RF/GPS Blocks/GPS Channel  Rice_Seed=Rice_Seeds(3)  tau_delay=taus_delay(3)  AWGN_Seed=AWGN_Seeds(3)  d=d(3)  tau=taus(3)
  GPS Channel3 : RF/GPS Blocks/GPS Channel  Rice_Seed=Rice_Seeds(4)  tau_delay=taus_delay(4)  AWGN_Seed=AWGN_Seeds(4)  d=d(4)  tau=taus(4)
  GPS Channel4 : RF/GPS Blocks/GPS Channel  Rice_Seed=Rice_Seeds(5)  tau_delay=taus_delay(5)  AWGN_Seed=AWGN_Seeds(5)  d=d(5)  tau=taus(5)
  GPS Channel5 : RF/GPS Blocks/GPS Channel  Rice_Seed=Rice_Seeds(6)  tau_delay=taus_delay(6)  AWGN_Seed=AWGN_Seeds(6)  d=d(6)  tau=taus(6)
  GPS Transmitter : RF/GPS Blocks/GPS Transmitter  tsrf=-1  CA_ID=CA(1)  P_Seed=P(1)
  GPS Transmitter1 : RF/GPS Blocks/GPS Transmitter  tsrf=-1  CA_ID=CA(2)  P_Seed=P(2)
  GPS Transmitter2 : RF/GPS Blocks/GPS Transmitter  tsrf=-1  CA_ID=CA(3)  P_Seed=P(3)
  GPS Transmitter3 : RF/GPS Blocks/GPS Transmitter  tsrf=-1  CA_ID=CA(3)  P_Seed=P(3)
  GPS Transmitter4 : RF/GPS Blocks/GPS Transmitter  tsrf=-1  CA_ID=CA(4)  P_Seed=P(4)
  GPS Transmitter5 : RF/GPS Blocks/GPS Transmitter  tsrf=-1  CA_ID=CA(5)  P_Seed=P(5)
  Navigation Data : RF/GPS Blocks/Navigation Data  Seed=Seeds(1)
  Navigation Data1 : RF/GPS Blocks/Navigation Data  Seed=Seeds(2)
  Navigation Data2 : RF/GPS Blocks/Navigation Data  Seed=Seeds(3)
  Navigation Data3 : RF/GPS Blocks/Navigation Data  Seed=Seeds(4)
  Navigation Data4 : RF/GPS Blocks/Navigation Data  Seed=Seeds(5)
  Navigation Data5 : RF/GPS Blocks/Navigation Data  Seed=Seeds(6)
  Sum : Sum  Inputs=++++++  SaturateOnIntegerOverflow=on
  Out1 : Outport  Port=1  InitialOutput=0
  wires:
  GPS Channel3/1 -> Sum/4
  GPS Channel4/1 -> Sum/5
  GPS Channel5/1 -> Sum/6
  GPS Channel2/1 -> Sum/3
  GPS Channel1/1 -> Sum/2
  GPS Channel/1 -> Sum/1
  Sum/1 -> Out1/1
  GPS Transmitter4/1 -> GPS Channel4/1
  Navigation Data4/1 -> GPS Transmitter4/1
  GPS Transmitter5/1 -> GPS Channel5/1
  Navigation Data5/1 -> GPS Transmitter5/1
  GPS Transmitter/1 -> GPS Channel/1
  Navigation Data/1 -> GPS Transmitter/1
  GPS Transmitter1/1 -> GPS Channel1/1
  Navigation Data1/1 -> GPS Transmitter1/1
  GPS Transmitter2/1 -> GPS Channel2/1
  Navigation Data2/1 -> GPS Transmitter2/1
  GPS Transmitter3/1 -> GPS Channel3/1
  Navigation Data3/1 -> GPS Transmitter3/1

== system RF/GPS Blocks/Direct Conversion Receiver ==
  note: Direct Conversion
  RF In : Inport  Port=1
  5th Order Decimation Filter : RF/A//D Blocks/5th Order Decimation Filter  N=32  fs=1E6
  5th Order Decimation Filter1 : RF/A//D Blocks/5th Order Decimation Filter  N=32  fs=1E6
  Butterworth LP Filter with Mismatch : RF/Filters/Butterworth LP Filter with Mismatch  w0=100*2*pi  order=4  ErrorStd=1
  Butterworth LP Filter with Mismatch1 : RF/Filters/Butterworth LP Filter with Mismatch  w0=100*2*pi  order=4  ErrorStd=1
  Fourth Order Sigma Delta with Mismatch : RF/A//D Blocks/Fourth Order Sigma Delta with Mismatch  NTF_Poles=p  NTF_Zeros=z  STF_Zeros=[inf inf inf]  STF_Gain=0.85  ErrorStd=1  fs=64E6
  Fourth Order Sigma Delta with Mismatch1 : RF/A//D Blocks/Fourth Order Sigma Delta with Mismatch  NTF_Poles=p  NTF_Zeros=z  STF_Zeros=[inf inf inf]  STF_Gain=0.85  ErrorStd=1  fs=64E6
  Join : dspcmplx/Join
  Non-Ideal Mixer : RF/Circuit Models/Non-Ideal Mixer  Gain1=0  IIP2=40  IIP3=40  fmax=1200  V1dB=-4  AWGNVRMS=1E-12  SeedAWGN=1  Fseed=2  f0=1000  N0=1.147E-7  fm=10E3  numtaps=100
  Non-Ideal Mixer1 : RF/Circuit Models/Non-Ideal Mixer  Gain1=0  IIP2=40  IIP3=40  fmax=1200  V1dB=-4  AWGNVRMS=1E-12  SeedAWGN=1  Fseed=2  f0=1000  N0=1.147E-7  fm=10E3  numtaps=100
  Non-Ideal  LNA : RF/Circuit Models/Non-Ideal  LNA  Gain1=0  IIP2=30  IIP3=20  AWGNVRMS=1E-3  fmax=3E9  V1dB=-4  SeedAWGN=123  FSeed=2  f0=1000  N0=1.147E-7  fm=10E3  numtaps=100
  Quadrature Oscillator : RF/Circuit Models/Quadrature Oscillator  PhiE=deg2rad(2)  AE=adb(0.1)  Phi=0  A=1  f0=1575.42E6
  RF Filter : RF/Filters/RF Filter  Q=5  f0=1575.42E6  n=1  Gi=1
  Data Out : Outport  Port=1  InitialOutput=0
  wires:
  Non-Ideal  LNA/1 -> Non-Ideal Mixer/2, Non-Ideal Mixer1/1
  RF Filter/1 -> Non-Ideal  LNA/1
  RF In/1 -> RF Filter/1
  Non-Ideal Mixer/1 -> Butterworth LP Filter with Mismatch/1
  Butterworth LP Filter with Mismatch/1 -> Fourth Order Sigma Delta with Mismatch/1
  Fourth Order Sigma Delta with Mismatch/1 -> 5th Order Decimation Filter/1
  Non-Ideal Mixer1/1 -> Butterworth LP Filter with Mismatch1/1
  Fourth Order Sigma Delta with Mismatch1/1 -> 5th Order Decimation Filter1/1
  Butterworth LP Filter with Mismatch1/1 -> Fourth Order Sigma Delta with Mismatch1/1
  5th Order Decimation Filter/1 -> Join/1
  5th Order Decimation Filter1/1 -> Join/2
  Join/1 -> Data Out/1
  Quadrature Oscillator/1 -> Non-Ideal Mixer/1
  Quadrature Oscillator/2 -> Non-Ideal Mixer1/2

== system RF/GPS Blocks/GPS Channel ==
  note: GPS Transmission Channel
  RF In : Inport  Port=1
  AWGN channel : Subsystem  mask(AWGN channel, fixed parameter){m=AWGN_Mean, d=AWGN_Variance, s=AWGN_Seed}
      mask prompts: m "Mean value:"; d "Variance (std^2):"; s "Initial Seed:"
      mask help: Additive white Gaussian noise channel with fixed mean and variance.
      settings: RTWFcnNameOpts=Auto  RTWFileNameOpts=Auto
      mask Help: This block adds white Gaussian noise to the input signal. The mean and the variance can be a scalar or vector with the same length as the input signal.
      mask Display:
      | plot(0,0,100,100,[05 15 10 10 05 10 18 14 13 7.5 13 41 44 47 50 53 57 59 100-[13 7.5 13 14 18 10 5 10 10 15 5]],[70 70 70 85 92 85 79 82 90 88.5 90 90 87 93 87 93 87 90 90 88.5 90 82 79 85 92 85 70 70 70]);
      | disp('AWGN')
  Atmospheric Delay : TransportDelay  DelayTime=tau  InitialInput=0  BufferSize=1024  PadeOrder=0
  Doppler and  Multi-path Fading : RF/Transmission  Channel Blocks/Doppler and  Multi-path Fading  seed=Rice_Seed  sigma=Rice_Sigma  K=Rice_K  DelaySpread=tau_delay
  Exponential Path Loss and Log-Normal Shadowing : RF/Transmission  Channel Blocks/Exponential Path Loss and Log-Normal Shadowing  d0=d_ref  d=d  p0=v_ref  Sigma_P=sigma_signal  n=n
  Impulse Noise : RF/Transmission  Channel Blocks/Impulse Noise  P_Impulse=Pulse_Prob  T_Impulse=Pulse_Duration  Amp_Var=Pulse_Sigma  Amp_Mean=Pulse_Amp  Num=Pulse_Poles  Denom=Pulse_Zeros
  Sum : Sum  Inputs=++  SaturateOnIntegerOverflow=on
  RF Out : Outport  Port=1  InitialOutput=0
  wires:
  Atmospheric Delay/1 -> Exponential Path Loss and Log-Normal Shadowing/1
  RF In/1 -> Atmospheric Delay/1
  AWGN channel/1(out_1) -> Sum/1
  Sum/1 -> RF Out/1
  Impulse Noise/1 -> Sum/2
  Exponential Path Loss and Log-Normal Shadowing/1 -> Doppler and  Multi-path Fading/1
  Doppler and  Multi-path Fading/1 -> AWGN channel/1(in_1)

== system RF/GPS Blocks/GPS Transmitter ==
  note: GPS Transmitter
  Data In : Inport  Port=1
  "BPSK mod, 1575MHz1" : Subsystem  mask(Passband MPSK modulation, modified.){M=2, td=1/10.23E6, Fc=1575.42E6, Ph=-pi/2, ts=tsrf}
      mask prompts: M "M-ary number (input integer in range [0, M-1]):"; td "Symbol interval (sec):"; Fc "Carrier frequency (Hz):"; Ph "Initial phase (rad):"; ts "Sample time (sec):"
      mask help: Modulate the input signal using M-ary phase shift keying method.
      settings: RTWFcnNameOpts=Auto  RTWFileNameOpts=Auto
      mask Help:
      | This block modulates a digital signal with a given carrier frequency using MPSK method. The inputs are integers in the range [0, M-1], where M is the M-ary number. When the symbol interval is a two element vector, the second element is the offset (default 0). The block keeps the input value at the offset time point for the entire interval.  The sample time, which was ignored by
      | MathWorks, now actually sets the sample time.
      mask Display:
      | plot(0,0,100,100,[5+15*[0 1 1 2 2 3] 50 50 50 50+1.5*[[0:.8:10] [10:.8:20] [20:.8:30]]],[85+8*[1 1 -1 -1 1 1] 85 99 75 85+10*[sin([0:.8:10]*pi*2/5) sin([10:.8:20]*pi*2/5 - pi) sin([20:.8:30]*pi*2/5)]]);
      | disp('BPSK')
  "BPSK mod, 1575MHz2" : Subsystem  mask(Passband MPSK modulation, modified.){M=2, td=1/10.23E6, Fc=1575.42E6, Ph=-pi, ts=tsrf}
      mask prompts: M "M-ary number (input integer in range [0, M-1]):"; td "Symbol interval (sec):"; Fc "Carrier frequency (Hz):"; Ph "Initial phase (rad):"; ts "Sample time (sec):"
      mask help: Modulate the input signal using M-ary phase shift keying method.
      settings: RTWFcnNameOpts=Auto  RTWFileNameOpts=Auto
      mask Help:
      | This block modulates a digital signal with a given carrier frequency using MPSK method. The inputs are integers in the range [0, M-1], where M is the M-ary number. When the symbol interval is a two element vector, the second element is the offset (default 0). The block keeps the input value at the offset time point for the entire interval.  The sample time, which was ignored by
      | MathWorks, now actually sets the sample time.
      mask Display:
      | plot(0,0,100,100,[5+15*[0 1 1 2 2 3] 50 50 50 50+1.5*[[0:.8:10] [10:.8:20] [20:.8:30]]],[85+8*[1 1 -1 -1 1 1] 85 99 75 85+10*[sin([0:.8:10]*pi*2/5) sin([10:.8:20]*pi*2/5 - pi) sin([20:.8:30]*pi*2/5)]]);
      | disp('BPSK')
  "C/A Code, 1.023MHz" : RF/GPS Blocks/C//A Code, 1.023MHz  CA_PRN_ID=CA_ID
  Gain : Gain  Gain=1/sqrt(2)  Multiplication=Element-wise(K.*u)  SaturateOnIntegerOverflow=on
  "P Code, 10.23MHz" : Subsystem  mask(P Sequence){P_Seed=P_Seed}
      mask prompts: P_Seed "Seed"
      mask help: Random sequence approximating GPS P sequence
      mask init:
      | [x,y]=srcsicon(5);
      settings: RTWFcnNameOpts=Auto  RTWFileNameOpts=Auto
      mask Help: Random sequence approximating the GPS P sequence, which is very long and not recreated in a commercial receiver.  Data rate is 10.23 MHz.
      mask Display: plot(0,0,100,100,x,y);disp('P Sequence ')
  Sum : Sum  Inputs=++  SaturateOnIntegerOverflow=on
  X (Mod 2) : Logic  Operator=XOR  Inputs=2
  X (Mod 2)1 : Logic  Operator=XOR  Inputs=2
  "L1 Out " : Outport  Port=1  InitialOutput=0
  wires:
  "BPSK mod, 1575MHz2"/1(out_1) -> Sum/2
  Gain/1 -> Sum/1
  X (Mod 2)1/1 -> "BPSK mod, 1575MHz2"/1(in_1)
  X (Mod 2)/1 -> "BPSK mod, 1575MHz1"/1(in_1)
  "BPSK mod, 1575MHz1"/1(out_1) -> Gain/1
  Sum/1 -> "L1 Out "/1
  Data In/1 -> X (Mod 2)1/1, X (Mod 2)/1
  "C/A Code, 1.023MHz"/1 -> X (Mod 2)1/2
  "P Code, 10.23MHz"/1(Out1) -> X (Mod 2)/2

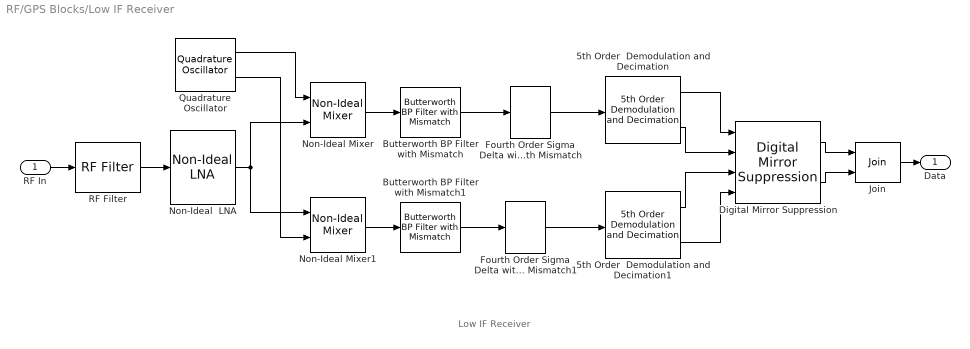
== system RF/GPS Blocks/Low IF Receiver ==
  note: Low IF Receiver
  RF In : Inport  Port=1
  5th Order  Demodulation and Decimation : RF/A//D Blocks/5th Order  Demodulation and Decimation  fs=10E6  fIF=3.75E6  N=25
  5th Order  Demodulation and Decimation1 : RF/A//D Blocks/5th Order  Demodulation and Decimation  fs=10E6  fIF=3.75E6  N=25
  Butterworth BP Filter with Mismatch : RF/Filters/Butterworth BP Filter with Mismatch  w1=200*2*pi  w2=300*2*pi  order=4  ErrorStd=1
  Butterworth BP Filter with Mismatch1 : RF/Filters/Butterworth BP Filter with Mismatch  w1=200*2*pi  w2=300*2*pi  order=4  ErrorStd=1
  Digital Mirror Suppression : RF/A//D Blocks/Digital Mirror Suppression  S=Signal Lower than LO
  Fourth Order Sigma Delta with Mismatch : RF/A//D Blocks/Fourth Order Sigma Delta with Mismatch  NTF_Poles=p  NTF_Zeros=z  STF_Zeros=[inf inf inf]  STF_Gain=0.85  ErrorStd=1  fs=64E6
  Fourth Order Sigma Delta with Mismatch1 : RF/A//D Blocks/Fourth Order Sigma Delta with Mismatch  NTF_Poles=p  NTF_Zeros=z  STF_Zeros=[inf inf inf]  STF_Gain=0.85  ErrorStd=1  fs=64E6
  Join : dspcmplx/Join
  Non-Ideal Mixer : RF/Circuit Models/Non-Ideal Mixer  Gain1=0  IIP2=40  IIP3=40  fmax=2*48E6  V1dB=-4  AWGNVRMS=1E-12  SeedAWGN=1  Fseed=2  f0=1000  N0=1.147E-7  fm=10E3  numtaps=100
  Non-Ideal Mixer1 : RF/Circuit Models/Non-Ideal Mixer  Gain1=0  IIP2=40  IIP3=40  fmax=2*48E6  V1dB=-4  AWGNVRMS=1E-12  SeedAWGN=1  Fseed=2  f0=1000  N0=1.147E-7  fm=10E3  numtaps=100
  Non-Ideal  LNA : RF/Circuit Models/Non-Ideal  LNA  Gain1=0  IIP2=30  IIP3=20  AWGNVRMS=1E-3  fmax=3E9  V1dB=-4  SeedAWGN=123  FSeed=2  f0=1000  N0=1.147E-7  fm=10E3  numtaps=100
  Quadrature Oscillator : RF/Circuit Models/Quadrature Oscillator  PhiE=deg2rad(2)  AE=adb(0.1)  Phi=0  A=1  f0=1575.42E6
  RF Filter : RF/Filters/RF Filter  Q=5  f0=1575.42E6  n=1  Gi=1
  Data : Outport  Port=1  InitialOutput=0
  wires:
  Butterworth BP Filter with Mismatch/1 -> Fourth Order Sigma Delta with Mismatch/1
  Fourth Order Sigma Delta with Mismatch/1 -> 5th Order  Demodulation and Decimation/1
  Fourth Order Sigma Delta with Mismatch1/1 -> 5th Order  Demodulation and Decimation1/1
  Butterworth BP Filter with Mismatch1/1 -> Fourth Order Sigma Delta with Mismatch1/1
  5th Order  Demodulation and Decimation/1 -> Digital Mirror Suppression/1
  5th Order  Demodulation and Decimation/2 -> Digital Mirror Suppression/2
  5th Order  Demodulation and Decimation1/1 -> Digital Mirror Suppression/3
  5th Order  Demodulation and Decimation1/2 -> Digital Mirror Suppression/4
  Digital Mirror Suppression/1 -> Join/1
  Join/1 -> Data/1
  Digital Mirror Suppression/2 -> Join/2
  Non-Ideal Mixer1/1 -> Butterworth BP Filter with Mismatch1/1
  Non-Ideal Mixer/1 -> Butterworth BP Filter with Mismatch/1
  Non-Ideal  LNA/1 -> Non-Ideal Mixer/2, Non-Ideal Mixer1/1
  RF Filter/1 -> Non-Ideal  LNA/1
  RF In/1 -> RF Filter/1
  Quadrature Oscillator/1 -> Non-Ideal Mixer/1
  Quadrature Oscillator/2 -> Non-Ideal Mixer1/2
